simulink model "CSTR_INOUT"  (Simulink 6.0)
settings: Solver=ode45  StartTime=0  StopTime=10  RelTol=1e-3
settings Model: LastModifiedBy=Larry  BufferReuse=off
settings DataIOCC: InitialState=[311.267; 8.5695]  SignalLoggingName=logsOut
settings OptimizationCC: BooleanDataType=off  InlineParams=on  BufferReuse=off
settings DebuggingCC: CheckExecutionContextPreStartOutputMsg=on  CheckExecutionContextRuntimeOutputMsg=on  SolverPrmCheckMsg=none
settings HardwareCC: TargetUnknown=on

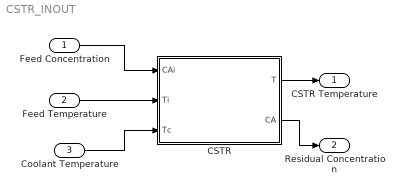
== system CSTR_INOUT ==
  Feed Concentration : Inport  Port=1  LatchInput=off
  Feed Temperature : Inport  Port=2  LatchInput=off
  Coolant Temperature : Inport  Port=3  LatchInput=off
  CSTR : Subsystem
  CSTR Temperature : Outport
  "Residual Concentration " : Outport  Port=2
  wires:
  Feed Temperature/1 -> CSTR/2(Ti)
  CSTR/1(T) -> CSTR Temperature/1
  Feed Concentration/1 -> CSTR/1(CAi)
  CSTR/2(CA) -> "Residual Concentration "/1
  Coolant Temperature/1 -> CSTR/3(Tc)

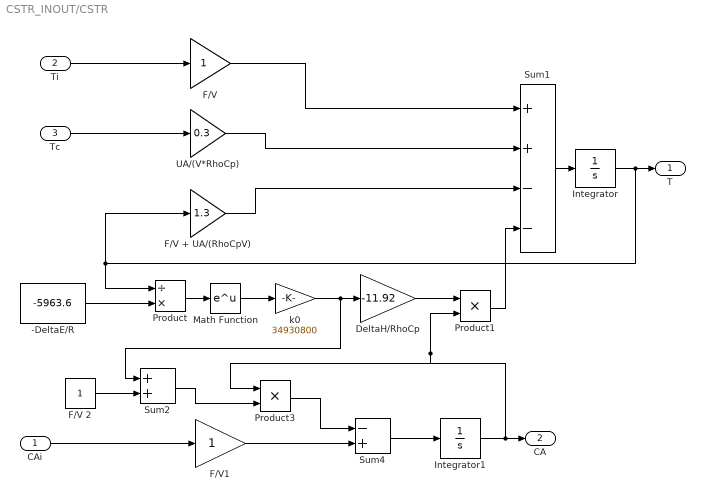
== system CSTR_INOUT/CSTR ==
  CAi : Inport  Port=1  LatchInput=off
  Ti : Inport  Port=2  LatchInput=off
  Tc : Inport  Port=3  LatchInput=off
  -DeltaE/R : Constant  Value=-5963.6
  DeltaH/RhoCp : Gain  Gain=-11.92  SaturateOnIntegerOverflow=on
  F/V : Gain  SaturateOnIntegerOverflow=on
  F/V + UA/(RhoCpV) : Gain  Gain=1.3  SaturateOnIntegerOverflow=on
  F/V 2 : Constant
  F/V1 : Gain  SaturateOnIntegerOverflow=on
  Integrator : Integrator  InitialCondition=311.267  LimitOutput=on  LowerSaturationLimit=0
  Integrator1 : Integrator  InitialCondition=8.5695  LimitOutput=on  LowerSaturationLimit=0
  Math Function : Math  SaturateOnIntegerOverflow=on
  Product : Product  Inputs=/*  SaturateOnIntegerOverflow=on  RndMeth=Zero  InputSameDT=on
  Product1 : Product  SaturateOnIntegerOverflow=on  RndMeth=Zero  InputSameDT=on
  Product3 : Product  SaturateOnIntegerOverflow=on  RndMeth=Zero  InputSameDT=on
  Sum1 : Sum  Inputs=++--  SaturateOnIntegerOverflow=on  InputSameDT=on
  Sum2 : Sum  SaturateOnIntegerOverflow=on  InputSameDT=on
  Sum4 : Sum  Inputs=-+  SaturateOnIntegerOverflow=on  InputSameDT=on
  UA/(V*RhoCp) : Gain  Gain=0.3  SaturateOnIntegerOverflow=on
  k0 : Gain  Gain=34930800  SaturateOnIntegerOverflow=on
  T : Outport
  CA : Outport  Port=2
  wires:
  F/V/1 -> Sum1/1
  Sum1/1 -> Integrator/1
  Integrator/1 -> Product/1, F/V + UA/(RhoCpV)/1, T/1
  UA/(V*RhoCp)/1 -> Sum1/2
  F/V + UA/(RhoCpV)/1 -> Sum1/3
  Product/1 -> Math Function/1
  Math Function/1 -> k0/1
  DeltaH/RhoCp/1 -> Product1/1
  Product1/1 -> Sum1/4
  k0/1 -> DeltaH/RhoCp/1, Sum2/1
  -DeltaE/R/1 -> Product/2
  Product3/1 -> Sum4/1
  Sum4/1 -> Integrator1/1
  Integrator1/1 -> Product3/1, Product1/2, CA/1
  F/V 2/1 -> Sum2/2
  F/V1/1 -> Sum4/2
  Ti/1 -> F/V/1
  CAi/1 -> F/V1/1
  Tc/1 -> UA/(V*RhoCp)/1
  Sum2/1 -> Product3/2
